simulink model "Copy_of_delay_plant_2015B"  (R2015b)
settings: Solver=VariableStepAuto  StartTime=0.0  StopTime=sim_run  FixedStep=0.0001  RelTol=1e-3
undefined symbols (not defined in the file): DiscIntNeverNeededParam, Standard_Devices, UDP_Protocol, zh_step
libraries: simulink x3, sldrtlib x2, dspnetwork x2
settings Model: Creator=Anony  LastModifiedBy=Anony

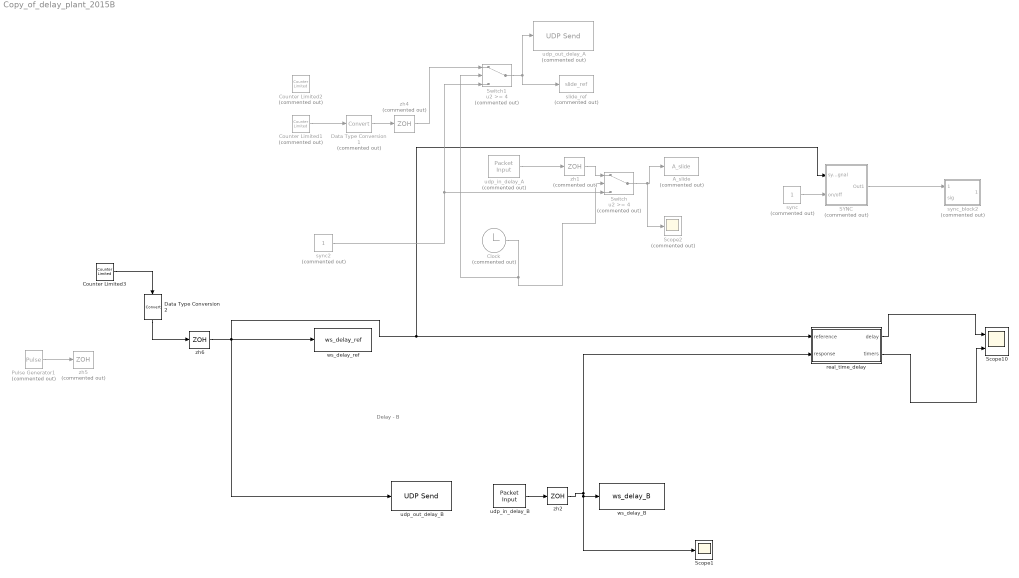
== system Copy_of_delay_plant_2015B ==
  note: Delay - B
  A_slide : ToWorkspace  Commented=on  VariableName=A_slide  SaveFormat=Timeseries  SampleTime=-1
  Clock : Clock  Commented=on
  Counter Limited1 : simulink/Sources/Counter Limited  Commented=on  uplimit=9  tsamp=0.1
  Counter Limited2 : simulink/Sources/Counter Limited  Commented=on  uplimit=999  tsamp=0.001
  Counter Limited3 : simulink/Sources/Counter Limited  uplimit=499  tsamp=0.001
  Data Type Conversion1 : DataTypeConversion  Commented=on
  Data Type Conversion2 : DataTypeConversion
  Pulse Generator1 : DiscretePulseGenerator  Commented=on  PulseType=Time based  Period=0.5  PulseWidth=0.1
  SYNC : Subsystem  Commented=on
  Scope1 : Scope
  Scope10 : Scope  NumInputPorts=2
  Scope2 : Scope  Commented=on
  Switch : Switch  Commented=on  Threshold=4
  Switch1 : Switch  Commented=on  Threshold=4
  real_time_delay : Subsystem
  slide_ref : ToWorkspace  Commented=on  VariableName=slide_ref  SaveFormat=Timeseries  SampleTime=-1
  sync : Constant  Commented=on
  sync2 : Constant  Commented=on
  sync_block2 : Subsystem  Commented=on
  udp_in_delay_A : sldrtlib/Packet Input  Commented=on  SampleTime=0.0001  MaxMissedTicks=inf  ShowMissedTicks=off  YieldWhenWaiting=off  DrvName=Standard_Devices/UDP_Protocol  DrvAddress=27000  DrvOptions=[2468394763 27000]  PacketSize=8  DataTypes='double'  ShowReady=off  ShowError=off  PacketID=1  ByteOrder=1  ShowTimestamp=off
      settings: AttributesFormatString=Standard Devices\nUDP Protocol [4E20h]
  udp_in_delay_B : sldrtlib/Packet Input  SampleTime=0.0001  MaxMissedTicks=inf  ShowMissedTicks=off  YieldWhenWaiting=off  DrvName=Standard_Devices/UDP_Protocol  DrvAddress=27010  DrvOptions=[2468394763 27010]  PacketSize=8  DataTypes='double'  ShowReady=off  ShowError=off  PacketID=1  ByteOrder=1  ShowTimestamp=off
      settings: AttributesFormatString=Standard Devices\nUDP Protocol [6982h]
  udp_out_delay_A : dspnetwork/UDP Send  Commented=on  remoteURL='147.32.183.11'  remotePort=28000  localURL='0.0.0.0'  localPortSource=Automatically determine  localPort=27000  sampletime=-1  separateLengthPort=0
  udp_out_delay_B : dspnetwork/UDP Send  remoteURL='147.32.183.11'  remotePort=28010  localURL='0.0.0.0'  localPortSource=Automatically determine  localPort=27000  sampletime=-1  separateLengthPort=0
  ws_delay_B : ToWorkspace  VariableName=ws_delay_B  SaveFormat=Timeseries  SampleTime=zh_step
  ws_delay_ref : ToWorkspace  VariableName=ws_delay_ref  SaveFormat=Timeseries  SampleTime=zh_step
  zh1 : ZeroOrderHold  Commented=on  SampleTime=0.001
  zh2 : ZeroOrderHold  SampleTime=zh_step
  zh4 : ZeroOrderHold  Commented=on  SampleTime=0.001
  zh5 : ZeroOrderHold  Commented=on  SampleTime=zh_step
  zh6 : ZeroOrderHold  SampleTime=0.001
  wires:
  udp_in_delay_B/1 -> zh2/1
  zh6/1 -> udp_out_delay_B/1, ws_delay_ref/1, real_time_delay/1(reference), SYNC/1(sync signal)
  zh2/1 -> Scope1/1, ws_delay_B/1, real_time_delay/2(response)
  real_time_delay/1(delay) -> Scope10/1
  real_time_delay/2(timers) -> Scope10/2
  udp_in_delay_A/1 -> zh1/1
  Counter Limited1/1 -> Data Type Conversion1/1
  zh1/1 -> Switch/1
  Data Type Conversion1/1 -> zh4/1
  SYNC/1(Out1) -> sync_block2/1(sync_sig)
  sync/1 -> SYNC/2(on/off)
  Clock/1 -> Switch/2, Switch1/2
  sync2/1 -> Switch1/3, Switch/3
  Switch/1 -> Scope2/1, A_slide/1
  Switch1/1 -> udp_out_delay_A/1, slide_ref/1
  zh4/1 -> Switch1/1
  Counter Limited3/1 -> Data Type Conversion2/1
  Pulse Generator1/1 -> zh5/1
  Data Type Conversion2/1 -> zh6/1

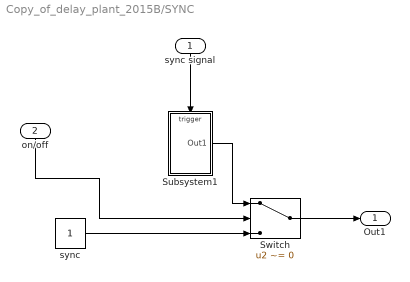
== system Copy_of_delay_plant_2015B/SYNC ==
  sync signal : Inport
  on/off : Inport  Port=2
  Subsystem1 : Subsystem
  Switch : Switch  Criteria=u2 ~= 0
  sync : Constant
  Out1 : Outport
  wires:
  sync/1 -> Switch/3
  sync signal/1 -> Subsystem1/Trigger
  Subsystem1/1(Out1) -> Switch/1
  Switch/1 -> Out1/1
  on/off/1 -> Switch/2

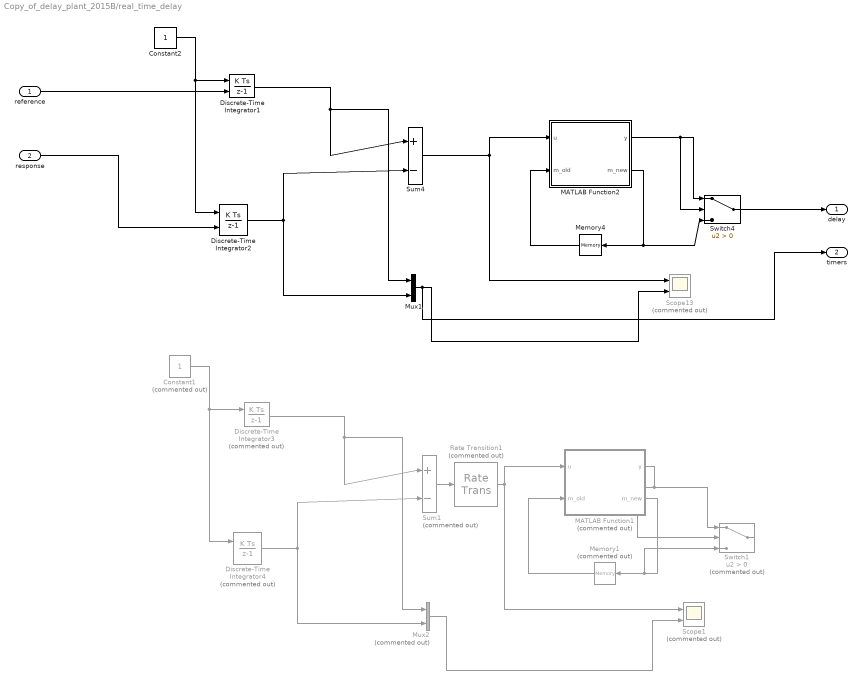
== system Copy_of_delay_plant_2015B/real_time_delay ==
  reference : Inport
  response : Inport  Port=2
  Constant1 : Constant  Commented=on
  Constant2 : Constant
  Discrete-Time Integrator1 : DiscreteIntegrator  ExternalReset=rising  InitialConditionSetting=State (most efficient)  SampleTime=0.001  ICPrevOutput=DiscIntNeverNeededParam  ICPrevScaledInput=DiscIntNeverNeededParam
  Discrete-Time Integrator2 : DiscreteIntegrator  ExternalReset=rising  InitialConditionSetting=State (most efficient)  SampleTime=0.001  ICPrevOutput=DiscIntNeverNeededParam  ICPrevScaledInput=DiscIntNeverNeededParam
  Discrete-Time Integrator3 : DiscreteIntegrator  Commented=on  ExternalReset=rising  InitialConditionSetting=State (most efficient)  SampleTime=0.001  ICPrevOutput=DiscIntNeverNeededParam  ICPrevScaledInput=DiscIntNeverNeededParam
  Discrete-Time Integrator4 : DiscreteIntegrator  Commented=on  ExternalReset=rising  InitialConditionSetting=State (most efficient)  SampleTime=0.001  ICPrevOutput=DiscIntNeverNeededParam  ICPrevScaledInput=DiscIntNeverNeededParam
  MATLAB Function1 : MATLAB Function  Commented=on  TreatAsAtomicUnit=on
  MATLAB Function2 : MATLAB Function  TreatAsAtomicUnit=on
  Memory1 : Memory  Commented=on
  Memory4 : Memory
  Mux1 : Mux  Inputs=2
  Mux2 : Mux  Commented=on  Inputs=2
  Rate Transition1 : RateTransition  Commented=on  OutPortSampleTimeOpt=Inherit
  Scope1 : Scope  Commented=on  NumInputPorts=2
  Scope13 : Scope  Commented=on  NumInputPorts=2
  Sum1 : Sum  Commented=on  Inputs=|+-
  Sum4 : Sum  Inputs=|+-
  Switch1 : Switch  Commented=on  Criteria=u2 > Threshold
  Switch4 : Switch  Criteria=u2 > Threshold
  delay : Outport
  timers : Outport  Port=2
  wires:
  Discrete-Time Integrator1/1 -> Mux1/1, Sum4/1
  reference/1 -> Discrete-Time Integrator1/2
  Constant2/1 -> Discrete-Time Integrator2/1, Discrete-Time Integrator1/1
  response/1 -> Discrete-Time Integrator2/2
  Switch4/1 -> delay/1
  MATLAB Function2/2(m_new) -> Memory4/1, Switch4/3
  Memory4/1 -> MATLAB Function2/2(m_old)
  Discrete-Time Integrator2/1 -> Mux1/2, Sum4/2
  Mux1/1 -> timers/1, Scope13/2
  MATLAB Function2/1(y) -> Switch4/2, Switch4/1
  Sum4/1 -> Scope13/1, MATLAB Function2/1(u)
  Discrete-Time Integrator3/1 -> Sum1/1, Mux2/1
  Constant1/1 -> Discrete-Time Integrator3/1, Discrete-Time Integrator4/1
  MATLAB Function1/2(m_new) -> Switch1/3, Memory1/1
  Sum1/1 -> Rate Transition1/1
  Memory1/1 -> MATLAB Function1/2(m_old)
  Discrete-Time Integrator4/1 -> Sum1/2, Mux2/2
  Mux2/1 -> Scope1/2
  MATLAB Function1/1(y) -> Switch1/1, Switch1/2
  Rate Transition1/1 -> MATLAB Function1/1(u), Scope1/1

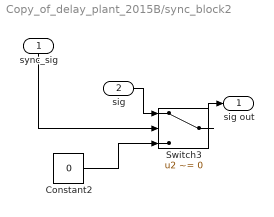
== system Copy_of_delay_plant_2015B/sync_block2 ==
  sync_sig : Inport
  sig : Inport  Port=2
  Constant2 : Constant  Value=0
  Switch3 : Switch  Criteria=u2 ~= 0
  sig out : Outport
  wires:
  Constant2/1 -> Switch3/3
  sig/1 -> Switch3/1
  Switch3/1 -> sig out/1
  sync_sig/1 -> Switch3/2

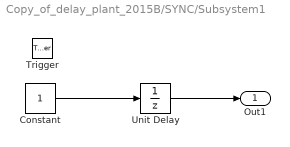
== system Copy_of_delay_plant_2015B/SYNC/Subsystem1 ==
  Trigger : TriggerPort  PortDimensions=1
  Constant : Constant
  Unit Delay : UnitDelay  SampleTime=-1
  Out1 : Outport
  wires:
  Unit Delay/1 -> Out1/1
  Constant/1 -> Unit Delay/1

== matlab function Copy_of_delay_plant_2015B/real_time_delay/MATLAB Function1 ==
  data: u input; y output; m_new output; m_old input
function [y,m_new] = fcn(u,m_old)
%#codegen
if(u>0)
    y = u;
    m_new = u;
else
    y =0;
    m_new = m_old;
end

== matlab function Copy_of_delay_plant_2015B/real_time_delay/MATLAB Function2 ==
  data: u input; y output; m_new output; m_old input
function [y,m_new] = fcn(u,m_old)
%#codegen
if(u>0)
    y = u;
    m_new = u;
else
    y =0;
    m_new = m_old;
end
